simulink model "Lab3ASimulinkOld"  (R2018a)
settings: Solver=VariableStepAuto  StartTime=0.0  StopTime=10.0  RelTol=1e-3
settings Model: Creator=rahul  LastModifiedBy=melab2

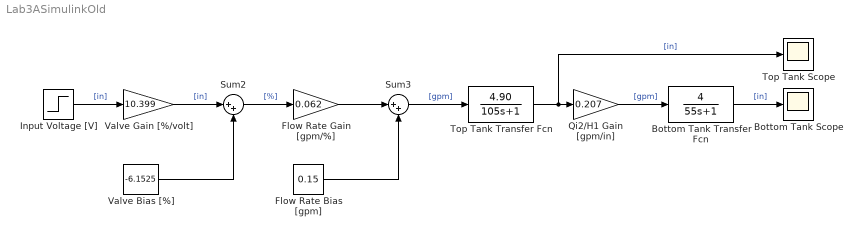
== system Lab3ASimulinkOld ==
  Bottom Tank Transfer Fcn : TransferFcn  Numerator=[4]  Denominator=[55 1]
  Bottom Tank Scope : Scope
  Flow Rate Bias [gpm] : Constant  Value=0.15
  Flow Rate Gain [gpm/%] : Gain  Gain=0.062
  Input Voltage [V] : Step  Time=0  Before=3.75  After=4  SampleTime=0
  Qi2/H1 Gain [gpm/in] : Gain  Gain=0.207
  Sum2 : Sum  Inputs=|++
  Sum3 : Sum  Inputs=|++
  Top Tank Transfer Fcn : TransferFcn  Numerator=[4.90]  Denominator=[105 1]
  Top Tank Scope : Scope
  Valve Bias [%] : Constant  Value=-6.1525
  Valve Gain [%/volt] : Gain  Gain=10.399
  wires:
  Flow Rate Gain [gpm/%]/1 -> Sum3/1
  Flow Rate Bias [gpm]/1 -> Sum3/2
  Valve Gain [%/volt]/1 -> Sum2/1  "[in]"
  Top Tank Transfer Fcn/1 -> Top Tank Scope/1, Qi2/H1 Gain [gpm/in]/1  "[in]"
  Sum3/1 -> Top Tank Transfer Fcn/1  "[gpm]"
  Bottom Tank Transfer Fcn/1 -> Bottom Tank Scope/1  "[in]"
  Input Voltage [V]/1 -> Valve Gain [%/volt]/1  "[in]"
  Qi2/H1 Gain [gpm/in]/1 -> Bottom Tank Transfer Fcn/1  "[gpm]"
  Sum2/1 -> Flow Rate Gain [gpm/%]/1  "[%]"
  Valve Bias [%]/1 -> Sum2/2
